simulink model "SecRwRtStHdrstUpwdDnwdIsPosChk"  (R2024b)
settings: Solver=FixedStepDiscrete  StartTime=0.0  StopTime=10.0  FixedStep=0.01  RelTol=1e-3
undefined symbols (not defined in the file or in its folder): KeSMSuSecRwStHeadrestUpwdDwnwdPosDelta_Val, KeSMSuSecRwStHeadrestUpwdDwnwdPosTolr_Val
libraries: StIsPosChkLib x9, simulink x5
settings Model: Creator=sn2xws  LastModifiedBy=sn55gm
settings Model: ModifiedHistory=|
  | 2023.8.1 V2.0.0 CR401790 增加模式21-26
  | V2.1.0
  | 2023.9.14  Bug 540886 修改模式判断到位的条件为10ms周期计算
  | Bug 541373 Md24到位置修改为常数1代表到位置
settings SolverCC: AlgebraicLoopSolver=TrustRegion
settings DataIOCC: SaveFormat=StructureWithTime  ReturnWorkspaceOutputs=off
settings OptimizationCC: DefaultParameterBehavior=Inlined  EnhancedBackFolding=on  PassReuseOutputArgsAs=Individual arguments  ZeroExternalMemoryAtStartup=off  ZeroInternalMemoryAtStartup=off  OptimizeBlockOrder=speed  DifferentSizesBufferReuse=on  OptimizationCustomize=off  EfficientTunableParamExpr=on
settings DebuggingCC: ParameterTunabilityLossMsg=error  UnconnectedInputMsg=warning  UnconnectedOutputMsg=warning  UnconnectedLineMsg=warning  ArithmeticOperatorsInVariantConditions=warning
settings ModelReferenceCC: EnableRefExpFcnMdlSchedulingChecks=on  ModelReferenceNumInstancesAllowed=Single
settings SFSimCC: MATLABDynamicMemAlloc=off  CustomCodeUndefinedFunction=UseInterfaceOnly
settings RTWCC: Description=AUTOSAR  SystemTargetFile=autosar.tlc  GenCodeOnly=on  TemplateMakefile=ert_default_tmf  GenerateReport=on  IncludeHyperlinkInReport=on  LaunchReport=on  DataTypeReplacement=CDataTypesFixedWidth  GenerateTraceInfo=on  GenerateTraceReport=on  GenerateTraceReportSl=on  GenerateTraceReportSf=on  GenerateTraceReportEml=on  GPUComputeCapability=3.5
settings CodeAppCC: ForceParamTrailComments=on  IgnoreCustomStorageClasses=off  OperatorAnnotations=on  SimulinkDataObjDesc=on  SFDataObjDesc=on  InsertBlockDesc=on
settings STFCustomTargetCC: TargetLangStandard=C99 (ISO)  MultiwordLength=256  ParMdlRefBuildCompliant=on  CompOptLevelCompliant=on  IncludeMdlTerminateFcn=off  CombineOutputUpdateFcns=on  SuppressErrorStatus=on  ERTCustomFileBanners=on  SupportNonFinite=off  SupportComplex=off  SupportContinuousTime=off  SupportNonInlinedSFcns=off  RemoveResetFunc=on  MATLABClassNameForMDSCustomization=Simulink.SoftwareTarget.ERTCustomization  AutosarCompliant=on  UseToolchainInfoCompliant=on  LookupTableObjectStructAxisOrder=2,1,3,4,...  LUTObjectStructOrderEvenSpacing=Size,Table,Breakpoints  SystemTargetFile=autosar.tlc
settings ERTTargetCC: TargetLangStandard=C99 (ISO)  ConcurrentExecutionCompliant=off  IncludeMdlTerminateFcn=off  SuppressErrorStatus=on  SupportNonFinite=off  SupportComplex=off  ModelStepFunctionPrototypeControlCompliant=off  CPPClassGenCompliant=off  AutosarCompliant=on  LookupTableObjectStructAxisOrder=2,1,3,4,...  LUTObjectStructOrderEvenSpacing=Size,Table,Breakpoints  ERTCustomFileTemplate=example_file_process.tlc  ERTFilePackagingFormat=Compact  BooleanTrueId=TRUE  BooleanFalseId=FALSE  DynamicArrayContainerType=coder::array

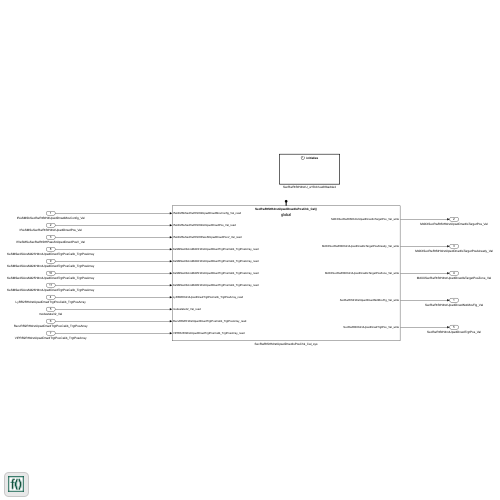
[thumbnail: Simulink's stored preview of the top-level diagram]
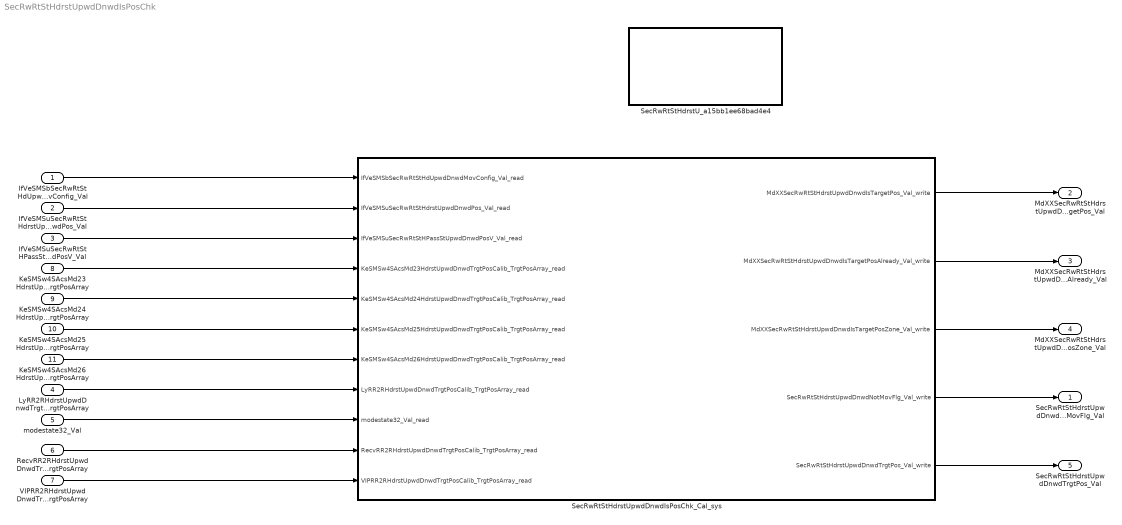
== system SecRwRtStHdrstUpwdDnwdIsPosChk ==
  IfVeSMSbSecRwRtStHdUpwdDnwdMovConfig_Val : Inport  OutDataTypeStr=boolean  PortDimensions=1
  IfVeSMSuSecRwRtStHdrstUpwdDnwdPos_Val : Inport  Port=2  OutDataTypeStr=uint16  PortDimensions=1
  IfVeSMSuSecRwRtStHPassStUpwdDnwdPosV_Val : Inport  Port=3  OutDataTypeStr=boolean  PortDimensions=1
  LyRR2RHdrstUpwdDnwdTrgtPosCalib_TrgtPosArray : Inport  Description=|  Port=4  OutDataTypeStr=uint16  PortDimensions=3
      | 0:Pos
      | 1:Max
      | 2:Min
  modestate32_Val : Inport  Port=5  OutDataTypeStr=uint32  PortDimensions=1
  RecvRR2RHdrstUpwdDnwdTrgtPosCalib_TrgtPosArray : Inport  Description=|  Port=6  OutDataTypeStr=uint16  PortDimensions=3
      | 0:Pos
      | 1:Max
      | 2:Min
  VIPRR2RHdrstUpwdDnwdTrgtPosCalib_TrgtPosArray : Inport  Description=|  Port=7  OutDataTypeStr=uint16  PortDimensions=3
      | 0:Pos
      | 1:Max
      | 2:Min
  KeSMSw4SAcsMd23HdrstUpwdDnwdTrgtPosCalib_TrgtPosArray : Inport  Description=|  Port=8  OutDataTypeStr=uint16  PortDimensions=3
      | 0:Pos
      | 1:Max
      | 2:Min
  KeSMSw4SAcsMd24HdrstUpwdDnwdTrgtPosCalib_TrgtPosArray : Inport  Description=|  Port=9  OutDataTypeStr=uint16  PortDimensions=3
      | 0:Pos
      | 1:Max
      | 2:Min
  KeSMSw4SAcsMd25HdrstUpwdDnwdTrgtPosCalib_TrgtPosArray : Inport  Description=|  Port=10  OutDataTypeStr=uint16  PortDimensions=3
      | 0:Pos
      | 1:Max
      | 2:Min
  KeSMSw4SAcsMd26HdrstUpwdDnwdTrgtPosCalib_TrgtPosArray : Inport  Description=|  Port=11  OutDataTypeStr=uint16  PortDimensions=3
      | 0:Pos
      | 1:Max
      | 2:Min
  SecRwRtStHdrstU_a15bb1ee68bad4e4 : Subsystem
  SecRwRtStHdrstUpwdDnwdIsPosChk_Cal_sys : Subsystem
  SecRwRtStHdrstUpwdDnwdNotMovFlg_Val : Outport  OutDataTypeStr=boolean  PortDimensions=1  VectorParamsAs1DForOutWhenUnconnected=off
  MdXXSecRwRtStHdrstUpwdDnwdIsTargetPos_Val : Outport  Port=2  OutDataTypeStr=uint32  PortDimensions=1  VectorParamsAs1DForOutWhenUnconnected=off
  MdXXSecRwRtStHdrstUpwdDnwdIsTargetPosAlready_Val : Outport  Port=3  OutDataTypeStr=uint32  PortDimensions=1  VectorParamsAs1DForOutWhenUnconnected=off
  MdXXSecRwRtStHdrstUpwdDnwdIsTargetPosZone_Val : Outport  Port=4  OutDataTypeStr=uint32  PortDimensions=1  VectorParamsAs1DForOutWhenUnconnected=off
  SecRwRtStHdrstUpwdDnwdTrgtPos_Val : Outport  Port=5  OutDataTypeStr=uint16  PortDimensions=1  VectorParamsAs1DForOutWhenUnconnected=off
  wires:
  IfVeSMSbSecRwRtStHdUpwdDnwdMovConfig_Val/1 -> SecRwRtStHdrstUpwdDnwdIsPosChk_Cal_sys/1(IfVeSMSbSecRwRtStHdUpwdDnwdMovConfig_Val_read)
  IfVeSMSuSecRwRtStHdrstUpwdDnwdPos_Val/1 -> SecRwRtStHdrstUpwdDnwdIsPosChk_Cal_sys/2(IfVeSMSuSecRwRtStHdrstUpwdDnwdPos_Val_read)
  IfVeSMSuSecRwRtStHPassStUpwdDnwdPosV_Val/1 -> SecRwRtStHdrstUpwdDnwdIsPosChk_Cal_sys/3(IfVeSMSuSecRwRtStHPassStUpwdDnwdPosV_Val_read)
  LyRR2RHdrstUpwdDnwdTrgtPosCalib_TrgtPosArray/1 -> SecRwRtStHdrstUpwdDnwdIsPosChk_Cal_sys/8(LyRR2RHdrstUpwdDnwdTrgtPosCalib_TrgtPosArray_read)
  modestate32_Val/1 -> SecRwRtStHdrstUpwdDnwdIsPosChk_Cal_sys/9(modestate32_Val_read)
  RecvRR2RHdrstUpwdDnwdTrgtPosCalib_TrgtPosArray/1 -> SecRwRtStHdrstUpwdDnwdIsPosChk_Cal_sys/10(RecvRR2RHdrstUpwdDnwdTrgtPosCalib_TrgtPosArray_read)
  VIPRR2RHdrstUpwdDnwdTrgtPosCalib_TrgtPosArray/1 -> SecRwRtStHdrstUpwdDnwdIsPosChk_Cal_sys/11(VIPRR2RHdrstUpwdDnwdTrgtPosCalib_TrgtPosArray_read)
  SecRwRtStHdrstUpwdDnwdIsPosChk_Cal_sys/1(MdXXSecRwRtStHdrstUpwdDnwdIsTargetPos_Val_write) -> MdXXSecRwRtStHdrstUpwdDnwdIsTargetPos_Val/1
  SecRwRtStHdrstUpwdDnwdIsPosChk_Cal_sys/2(MdXXSecRwRtStHdrstUpwdDnwdIsTargetPosAlready_Val_write) -> MdXXSecRwRtStHdrstUpwdDnwdIsTargetPosAlready_Val/1
  SecRwRtStHdrstUpwdDnwdIsPosChk_Cal_sys/3(MdXXSecRwRtStHdrstUpwdDnwdIsTargetPosZone_Val_write) -> MdXXSecRwRtStHdrstUpwdDnwdIsTargetPosZone_Val/1
  SecRwRtStHdrstUpwdDnwdIsPosChk_Cal_sys/4(SecRwRtStHdrstUpwdDnwdNotMovFlg_Val_write) -> SecRwRtStHdrstUpwdDnwdNotMovFlg_Val/1
  SecRwRtStHdrstUpwdDnwdIsPosChk_Cal_sys/5(SecRwRtStHdrstUpwdDnwdTrgtPos_Val_write) -> SecRwRtStHdrstUpwdDnwdTrgtPos_Val/1
  KeSMSw4SAcsMd23HdrstUpwdDnwdTrgtPosCalib_TrgtPosArray/1 -> SecRwRtStHdrstUpwdDnwdIsPosChk_Cal_sys/4(KeSMSw4SAcsMd23HdrstUpwdDnwdTrgtPosCalib_TrgtPosArray_read)
  KeSMSw4SAcsMd24HdrstUpwdDnwdTrgtPosCalib_TrgtPosArray/1 -> SecRwRtStHdrstUpwdDnwdIsPosChk_Cal_sys/5(KeSMSw4SAcsMd24HdrstUpwdDnwdTrgtPosCalib_TrgtPosArray_read)
  KeSMSw4SAcsMd25HdrstUpwdDnwdTrgtPosCalib_TrgtPosArray/1 -> SecRwRtStHdrstUpwdDnwdIsPosChk_Cal_sys/6(KeSMSw4SAcsMd25HdrstUpwdDnwdTrgtPosCalib_TrgtPosArray_read)
  KeSMSw4SAcsMd26HdrstUpwdDnwdTrgtPosCalib_TrgtPosArray/1 -> SecRwRtStHdrstUpwdDnwdIsPosChk_Cal_sys/7(KeSMSw4SAcsMd26HdrstUpwdDnwdTrgtPosCalib_TrgtPosArray_read)

== system SecRwRtStHdrstUpwdDnwdIsPosChk/SecRwRtStHdrstU_a15bb1ee68bad4e4 ==
  Event Listener : EventListener  EventName=reset

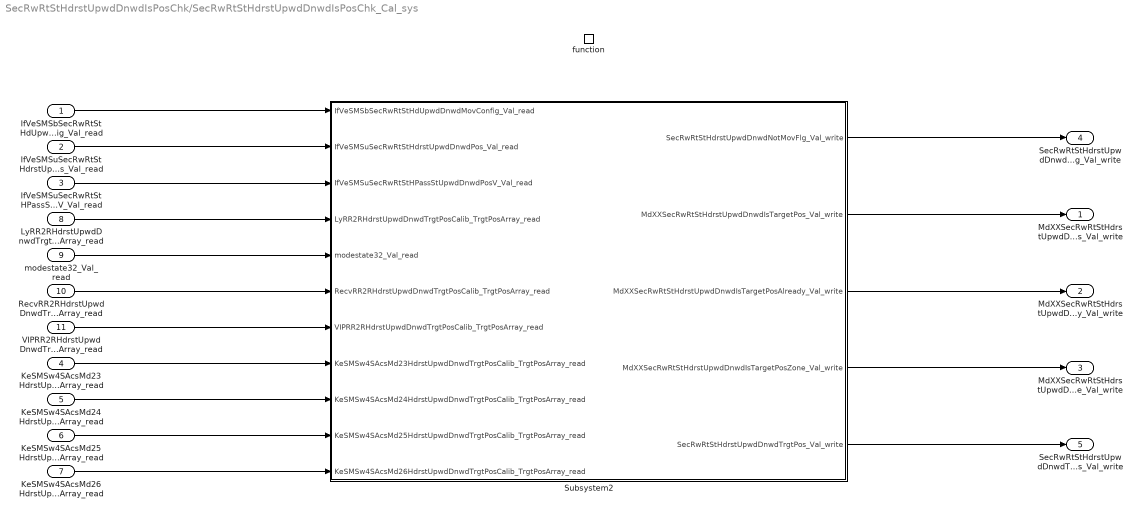
== system SecRwRtStHdrstUpwdDnwdIsPosChk/SecRwRtStHdrstUpwdDnwdIsPosChk_Cal_sys ==
  IfVeSMSbSecRwRtStHdUpwdDnwdMovConfig_Val_read : Inport
  IfVeSMSuSecRwRtStHdrstUpwdDnwdPos_Val_read : Inport  Port=2
  IfVeSMSuSecRwRtStHPassStUpwdDnwdPosV_Val_read : Inport  Port=3
  KeSMSw4SAcsMd23HdrstUpwdDnwdTrgtPosCalib_TrgtPosArray_read : Inport  Port=4
  KeSMSw4SAcsMd24HdrstUpwdDnwdTrgtPosCalib_TrgtPosArray_read : Inport  Port=5
  KeSMSw4SAcsMd25HdrstUpwdDnwdTrgtPosCalib_TrgtPosArray_read : Inport  Port=6
  KeSMSw4SAcsMd26HdrstUpwdDnwdTrgtPosCalib_TrgtPosArray_read : Inport  Port=7
  LyRR2RHdrstUpwdDnwdTrgtPosCalib_TrgtPosArray_read : Inport  Port=8
  modestate32_Val_read : Inport  Port=9
  RecvRR2RHdrstUpwdDnwdTrgtPosCalib_TrgtPosArray_read : Inport  Port=10
  VIPRR2RHdrstUpwdDnwdTrgtPosCalib_TrgtPosArray_read : Inport  Port=11
  function : TriggerPort  TriggerType=function-call  IsSimulinkFunction=on  FunctionName=SecRwRtStHdrstUpwdDnwdIsPosChk_Cal  VariantControl=(inherit)
  Subsystem2 : Subsystem
  MdXXSecRwRtStHdrstUpwdDnwdIsTargetPos_Val_write : Outport  VectorParamsAs1DForOutWhenUnconnected=off
      settings: EnsureOutportIsVirtual=on
  MdXXSecRwRtStHdrstUpwdDnwdIsTargetPosAlready_Val_write : Outport  Port=2  VectorParamsAs1DForOutWhenUnconnected=off
      settings: EnsureOutportIsVirtual=on
  MdXXSecRwRtStHdrstUpwdDnwdIsTargetPosZone_Val_write : Outport  Port=3  VectorParamsAs1DForOutWhenUnconnected=off
      settings: EnsureOutportIsVirtual=on
  SecRwRtStHdrstUpwdDnwdNotMovFlg_Val_write : Outport  Port=4  VectorParamsAs1DForOutWhenUnconnected=off
      settings: EnsureOutportIsVirtual=on
  SecRwRtStHdrstUpwdDnwdTrgtPos_Val_write : Outport  Port=5  VectorParamsAs1DForOutWhenUnconnected=off
      settings: EnsureOutportIsVirtual=on
  wires:
  LyRR2RHdrstUpwdDnwdTrgtPosCalib_TrgtPosArray_read/1 -> Subsystem2/4(LyRR2RHdrstUpwdDnwdTrgtPosCalib_TrgtPosArray_read)
  modestate32_Val_read/1 -> Subsystem2/5(modestate32_Val_read)
  RecvRR2RHdrstUpwdDnwdTrgtPosCalib_TrgtPosArray_read/1 -> Subsystem2/6(RecvRR2RHdrstUpwdDnwdTrgtPosCalib_TrgtPosArray_read)
  VIPRR2RHdrstUpwdDnwdTrgtPosCalib_TrgtPosArray_read/1 -> Subsystem2/7(VIPRR2RHdrstUpwdDnwdTrgtPosCalib_TrgtPosArray_read)
  KeSMSw4SAcsMd23HdrstUpwdDnwdTrgtPosCalib_TrgtPosArray_read/1 -> Subsystem2/8(KeSMSw4SAcsMd23HdrstUpwdDnwdTrgtPosCalib_TrgtPosArray_read)
  IfVeSMSuSecRwRtStHPassStUpwdDnwdPosV_Val_read/1 -> Subsystem2/3(IfVeSMSuSecRwRtStHPassStUpwdDnwdPosV_Val_read)
  KeSMSw4SAcsMd24HdrstUpwdDnwdTrgtPosCalib_TrgtPosArray_read/1 -> Subsystem2/9(KeSMSw4SAcsMd24HdrstUpwdDnwdTrgtPosCalib_TrgtPosArray_read)
  KeSMSw4SAcsMd25HdrstUpwdDnwdTrgtPosCalib_TrgtPosArray_read/1 -> Subsystem2/10(KeSMSw4SAcsMd25HdrstUpwdDnwdTrgtPosCalib_TrgtPosArray_read)
  IfVeSMSuSecRwRtStHdrstUpwdDnwdPos_Val_read/1 -> Subsystem2/2(IfVeSMSuSecRwRtStHdrstUpwdDnwdPos_Val_read)
  KeSMSw4SAcsMd26HdrstUpwdDnwdTrgtPosCalib_TrgtPosArray_read/1 -> Subsystem2/11(KeSMSw4SAcsMd26HdrstUpwdDnwdTrgtPosCalib_TrgtPosArray_read)
  IfVeSMSbSecRwRtStHdUpwdDnwdMovConfig_Val_read/1 -> Subsystem2/1(IfVeSMSbSecRwRtStHdUpwdDnwdMovConfig_Val_read)
  Subsystem2/1(SecRwRtStHdrstUpwdDnwdNotMovFlg_Val_write) -> SecRwRtStHdrstUpwdDnwdNotMovFlg_Val_write/1
  Subsystem2/2(MdXXSecRwRtStHdrstUpwdDnwdIsTargetPos_Val_write) -> MdXXSecRwRtStHdrstUpwdDnwdIsTargetPos_Val_write/1
  Subsystem2/3(MdXXSecRwRtStHdrstUpwdDnwdIsTargetPosAlready_Val_write) -> MdXXSecRwRtStHdrstUpwdDnwdIsTargetPosAlready_Val_write/1
  Subsystem2/4(MdXXSecRwRtStHdrstUpwdDnwdIsTargetPosZone_Val_write) -> MdXXSecRwRtStHdrstUpwdDnwdIsTargetPosZone_Val_write/1
  Subsystem2/5(SecRwRtStHdrstUpwdDnwdTrgtPos_Val_write) -> SecRwRtStHdrstUpwdDnwdTrgtPos_Val_write/1

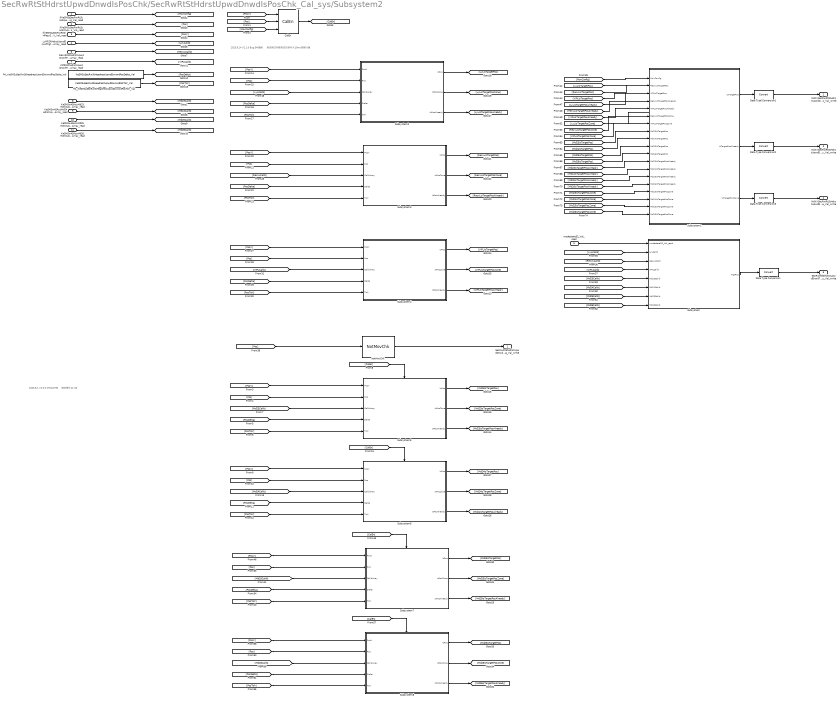
== system SecRwRtStHdrstUpwdDnwdIsPosChk/SecRwRtStHdrstUpwdDnwdIsPosChk_Cal_sys/Subsystem2 ==
  note: 2023.9.14 V2.1.0 Bug 540886 修改模式判断到位的条件为10ms周期计算
  note: 2023.8.1 V2.0.0 CR401790 增加模式21-26
  IfVeSMSbSecRwRtStHdUpwdDnwdMovConfig_Val_read : Inport
  IfVeSMSuSecRwRtStHdrstUpwdDnwdPos_Val_read : Inport  Port=2
  IfVeSMSuSecRwRtStHPassStUpwdDnwdPosV_Val_read : Inport  Port=3
  LyRR2RHdrstUpwdDnwdTrgtPosCalib_TrgtPosArray_read : Inport  Port=4
  modestate32_Val_read : Inport  Port=5
  RecvRR2RHdrstUpwdDnwdTrgtPosCalib_TrgtPosArray_read : Inport  Port=6
  VIPRR2RHdrstUpwdDnwdTrgtPosCalib_TrgtPosArray_read : Inport  Port=7
  KeSMSw4SAcsMd23HdrstUpwdDnwdTrgtPosCalib_TrgtPosArray_read : Inport  Port=8
  KeSMSw4SAcsMd24HdrstUpwdDnwdTrgtPosCalib_TrgtPosArray_read : Inport  Port=9
  KeSMSw4SAcsMd25HdrstUpwdDnwdTrgtPosCalib_TrgtPosArray_read : Inport  Port=10
  KeSMSw4SAcsMd26HdrstUpwdDnwdTrgtPosCalib_TrgtPosArray_read : Inport  Port=11
  CalEn : StIsPosChkLib/CalEn  SystemSampleTime=-1  VariantActivationTime=update diagram  AllowFlexibleInterface=on  Latency=0  AutoFrameSizeCalculation=off
  Data Type Conversion{,1..3} (4 alike) : DataTypeConversion  SaturateOnIntegerOverflow=off  RndMeth=Floor
  NotMovChk : StIsPosChkLib/NotMovChk  SystemSampleTime=-1  VariantActivationTime=update diagram  AllowFlexibleInterface=on  Latency=0  AutoFrameSizeCalculation=off
  PA_KeSMSuSecRwStHeadrestUpwdDwnwdPosDelta_Val : Constant  Value=KeSMSuSecRwStHeadrestUpwdDwnwdPosDelta_Val
  PA_KeSMSuSecRwStHeadrestUpwdDwnwdPosTolr_Val : Constant  Value=KeSMSuSecRwStHeadrestUpwdDwnwdPosTolr_Val
  Subsystem : Subsystem
  Subsystem1 : Subsystem
  Subsystem2 : Subsystem
  Subsystem3 : Subsystem
  Subsystem4 : Subsystem
  Subsystem5 : Subsystem
  Subsystem6 : Subsystem
  Subsystem7 : Subsystem
  Subsystem8 : Subsystem
  SecRwRtStHdrstUpwdDnwdNotMovFlg_Val_write : Outport  VectorParamsAs1DForOutWhenUnconnected=off
      settings: EnsureOutportIsVirtual=on
  MdXXSecRwRtStHdrstUpwdDnwdIsTargetPos_Val_write : Outport  Port=2  VectorParamsAs1DForOutWhenUnconnected=off
      settings: EnsureOutportIsVirtual=on
  MdXXSecRwRtStHdrstUpwdDnwdIsTargetPosAlready_Val_write : Outport  Port=3  VectorParamsAs1DForOutWhenUnconnected=off
      settings: EnsureOutportIsVirtual=on
  MdXXSecRwRtStHdrstUpwdDnwdIsTargetPosZone_Val_write : Outport  Port=4  VectorParamsAs1DForOutWhenUnconnected=off
      settings: EnsureOutportIsVirtual=on
  SecRwRtStHdrstUpwdDnwdTrgtPos_Val_write : Outport  Port=5  VectorParamsAs1DForOutWhenUnconnected=off
      settings: EnsureOutportIsVirtual=on
  wires:
  [VIPLIsTargetPosAlready] -> Subsystem1/5(VIPLIsTargetPosAlready)
  [Pos] -> NotMovChk/1
  PA_KeSMSuSecRwStHeadrestUpwdDwnwdPosTolr_Val/1 -> [PosTolr]
  [PosV] -> Subsystem2/1(PosV)
  [VIPLIsTargetPosZone] -> Subsystem1/7(VIPLIsTargetPosZone)
  modestate32_Val_read/1 -> Subsystem/1(modestate32_Val_read)
  NotMovChk/1 -> SecRwRtStHdrstUpwdDnwdNotMovFlg_Val_write/1
  Subsystem2/3(IsPosAlready) -> [LyLIsTargetPosAlready]
  [PosV] -> Subsystem3/1(PosV)
  [PosDelta] -> Subsystem3/4(Delta)
  [RecvLIsTargetPosZone] -> Subsystem1/6(RecvLIsTargetPosZone)
  Subsystem2/1(IsPos) -> [LyLIsTargetPos]
  [LyLIsTargetPosAlready] -> ?
  [PosDelta] -> Subsystem2/4(Delta)
  LyRR2RHdrstUpwdDnwdTrgtPosCalib_TrgtPosArray_read/1 -> [LyLCalib]
  RecvRR2RHdrstUpwdDnwdTrgtPosCalib_TrgtPosArray_read/1 -> [RecvLCalib]
  [PosV] -> Subsystem4/1(PosV)
  Subsystem4/2(IsPosZone) -> [VIPLIsTargetPosZone]
  Subsystem3/3(IsPosAlready) -> [RecvLIsTargetPosAlready]
  [VIPLCalib] -> Subsystem/4(VIPLCalib)
  [PosTolr] -> Subsystem3/5(Tolr)
  Data Type Conversion2/1 -> MdXXSecRwRtStHdrstUpwdDnwdIsTargetPosAlready_Val_write/1
  Subsystem1/1(IsTargetPos) -> Data Type Conversion1/1
  Subsystem4/1(IsPos) -> [VIPLIsTargetPos]
  VIPRR2RHdrstUpwdDnwdTrgtPosCalib_TrgtPosArray_read/1 -> [VIPLCalib]
  [Pos] -> Subsystem2/2(Pos)
  Subsystem3/2(IsPosZone) -> [RecvLIsTargetPosZone]
  PA_KeSMSuSecRwStHeadrestUpwdDwnwdPosDelta_Val/1 -> [PosDelta]
  [RecvLIsTargetPos] -> Subsystem1/2(RecvLIsTargetPos)
  Subsystem1/2(IsTargetPosAlready) -> Data Type Conversion2/1
  [LyLIsTargetPosZone] -> ?
  [PosTolr] -> Subsystem4/5(Tolr)
  CalEn/1 -> [CalEn]
  Subsystem/1(TrgtPos) -> Data Type Conversion/1
  Subsystem3/1(IsPos) -> [RecvLIsTargetPos]
  [RecvLCalib] -> Subsystem/3(RecvLCalib)
  [PosV] -> CalEn/1
  Subsystem4/3(IsPosAlready) -> [VIPLIsTargetPosAlready]
  [RecvLCalib] -> Subsystem3/3(CalibArray)
  Data Type Conversion1/1 -> MdXXSecRwRtStHdrstUpwdDnwdIsTargetPos_Val_write/1
  [MovConfig] -> Subsystem1/1(MovConfig)
  IfVeSMSuSecRwRtStHPassStUpwdDnwdPosV_Val_read/1 -> [PosV]
  [PosTolr] -> Subsystem2/5(Tolr)
  Subsystem2/2(IsPosZone) -> [LyLIsTargetPosZone]
  [Pos] -> Subsystem4/2(Pos)
  IfVeSMSbSecRwRtStHdUpwdDnwdMovConfig_Val_read/1 -> [MovConfig]
  [RecvLIsTargetPosAlready] -> Subsystem1/4(RecvLIsTargetPosAlready)
  Subsystem1/3(IsTargetPosZone) -> Data Type Conversion3/1
  [VIPLIsTargetPos] -> Subsystem1/3(VIPLIsTargetPos)
  [PosDelta] -> Subsystem4/4(Delta)
  [VIPLCalib] -> Subsystem4/3(CalibArray)
  [Pos] -> CalEn/2
  IfVeSMSuSecRwRtStHdrstUpwdDnwdPos_Val_read/1 -> [Pos]
  [LyLCalib] -> Subsystem2/3(CalibArray)
  [LyLCalib] -> Subsystem/2(LyLCalib)
  [Pos] -> Subsystem3/2(Pos)
  [MovConfig] -> CalEn/3
  Data Type Conversion3/1 -> MdXXSecRwRtStHdrstUpwdDnwdIsTargetPosZone_Val_write/1
  Data Type Conversion/1 -> SecRwRtStHdrstUpwdDnwdTrgtPos_Val_write/1
  [LyLIsTargetPos] -> ?
  KeSMSw4SAcsMd23HdrstUpwdDnwdTrgtPosCalib_TrgtPosArray_read/1 -> [Md23Calib]
  KeSMSw4SAcsMd24HdrstUpwdDnwdTrgtPosCalib_TrgtPosArray_read/1 -> [Md24Calib]
  KeSMSw4SAcsMd25HdrstUpwdDnwdTrgtPosCalib_TrgtPosArray_read/1 -> [Md25Calib]
  KeSMSw4SAcsMd26HdrstUpwdDnwdTrgtPosCalib_TrgtPosArray_read/1 -> [Md26Calib]
  [Md23Calib] -> Subsystem5/3(CalibArray)
  [PosDelta] -> Subsystem5/4(Delta)
  [Pos] -> Subsystem5/2(Pos)
  Subsystem5/3(IsPosAlready) -> [Md23IsTargetPosAlready]
  [PosTolr] -> Subsystem5/5(Tolr)
  Subsystem5/1(IsPos) -> [Md23IsTargetPos]
  Subsystem5/2(IsPosZone) -> [Md23IsTargetPosZone]
  [PosV] -> Subsystem5/1(PosV)
  [CalEn] -> Subsystem5/Enable
  [CalEn] -> Subsystem6/Enable
  [PosV] -> Subsystem6/1(PosV)
  Subsystem6/2(IsPosZone) -> [Md24IsTargetPosZone]
  Subsystem6/1(IsPos) -> [Md24IsTargetPos]
  [PosTolr] -> Subsystem6/5(Tolr)
  Subsystem6/3(IsPosAlready) -> [Md24IsTargetPosAlready]
  [Pos] -> Subsystem6/2(Pos)
  [PosDelta] -> Subsystem6/4(Delta)
  [Md24Calib] -> Subsystem6/3(CalibArray)
  [Md25Calib] -> Subsystem7/3(CalibArray)
  [PosDelta] -> Subsystem7/4(Delta)
  [Pos] -> Subsystem7/2(Pos)
  Subsystem7/3(IsPosAlready) -> [Md25IsTargetPosAlready]
  [PosTolr] -> Subsystem7/5(Tolr)
  Subsystem7/1(IsPos) -> [Md25IsTargetPos]
  Subsystem7/2(IsPosZone) -> [Md25IsTargetPosZone]
  [PosV] -> Subsystem7/1(PosV)
  [CalEn] -> Subsystem7/Enable
  [CalEn] -> Subsystem8/Enable
  [PosV] -> Subsystem8/1(PosV)
  Subsystem8/2(IsPosZone) -> [Md26IsTargetPosZone]
  Subsystem8/1(IsPos) -> [Md26IsTargetPos]
  [PosTolr] -> Subsystem8/5(Tolr)
  Subsystem8/3(IsPosAlready) -> [Md26IsTargetPosAlready]
  [Pos] -> Subsystem8/2(Pos)
  [PosDelta] -> Subsystem8/4(Delta)
  [Md26Calib] -> Subsystem8/3(CalibArray)
  [Md23Calib] -> Subsystem/5(Md23Calib)
  [Md24Calib] -> Subsystem/6(Md24Calib)
  [Md25Calib] -> Subsystem/7(Md25Calib)
  [Md26Calib] -> Subsystem/8(Md26Calib)
  [Md23IsTargetPos] -> Subsystem1/8(Md23IsTargetPos)
  [Md24IsTargetPos] -> Subsystem1/9(Md24IsTargetPos)
  [Md25IsTargetPos] -> Subsystem1/10(Md25IsTargetPos)
  [Md26IsTargetPos] -> Subsystem1/11(Md26IsTargetPos)
  [Md23IsTargetPosAlready] -> Subsystem1/12(Md23IsTargetPosAlready)
  [Md24IsTargetPosAlready] -> Subsystem1/13(Md24IsTargetPosAlready)
  [Md25IsTargetPosAlready] -> Subsystem1/14(Md25IsTargetPosAlready)
  [Md26IsTargetPosAlready] -> Subsystem1/15(Md26IsTargetPosAlready)
  [Md23IsTargetPosZone] -> Subsystem1/16(Md23IsTargetPosZone)
  [Md24IsTargetPosZone] -> Subsystem1/17(Md24IsTargetPosZone)
  [Md25IsTargetPosZone] -> Subsystem1/18(Md25IsTargetPosZone)
  [Md26IsTargetPosZone] -> Subsystem1/19(Md26IsTargetPosZone)

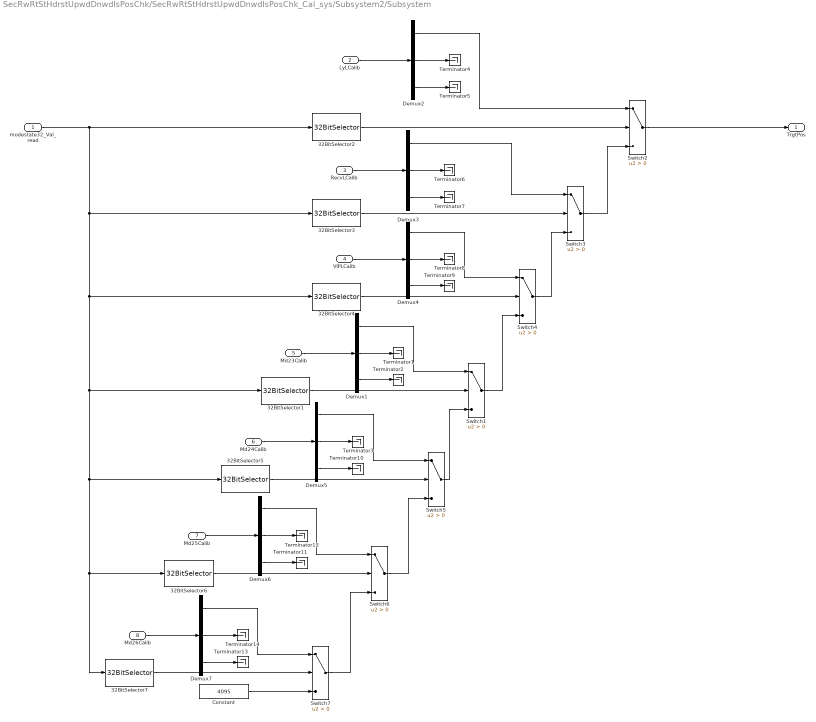
== system SecRwRtStHdrstUpwdDnwdIsPosChk/SecRwRtStHdrstUpwdDnwdIsPosChk_Cal_sys/Subsystem2/Subsystem ==
  modestate32_Val_read : Inport
  LyLCalib : Inport  Port=2
  RecvLCalib : Inport  Port=3
  VIPLCalib : Inport  Port=4
  Md23Calib : Inport  Port=5
  Md24Calib : Inport  Port=6
  Md25Calib : Inport  Port=7
  Md26Calib : Inport  Port=8
  32BitSelector1 : StIsPosChkLib/32BitSelector  BitNum=22
  32BitSelector2 : StIsPosChkLib/32BitSelector  BitNum=14
  32BitSelector3 : StIsPosChkLib/32BitSelector  BitNum=12
  32BitSelector4 : StIsPosChkLib/32BitSelector  BitNum=11
  32BitSelector5 : StIsPosChkLib/32BitSelector  BitNum=23
  32BitSelector6 : StIsPosChkLib/32BitSelector  BitNum=24
  32BitSelector7 : StIsPosChkLib/32BitSelector  BitNum=25
  Constant : Constant  Value=4095  OutDataTypeStr=uint16
  Demux{1..7} (7 alike) : Demux  Outputs=3
  Switch{1..7} (7 alike) : Switch  Criteria=u2 > Threshold  SaturateOnIntegerOverflow=off  InputSameDT=off
  Terminator{1..14} (14 alike) : Terminator
  TrgtPos : Outport  VectorParamsAs1DForOutWhenUnconnected=off
      settings: EnsureOutportIsVirtual=on
  wires:
  modestate32_Val_read/1 -> 32BitSelector2/1, 32BitSelector3/1, 32BitSelector7/1, 32BitSelector6/1, 32BitSelector5/1, 32BitSelector1/1, 32BitSelector4/1
  Switch2/1 -> TrgtPos/1
  Switch3/1 -> Switch2/3
  Switch4/1 -> Switch3/3
  32BitSelector2/1 -> Switch2/2
  32BitSelector3/1 -> Switch3/2
  32BitSelector4/1 -> Switch4/2
  Demux2/1 -> Switch2/1
  Demux2/3 -> Terminator5/1
  Demux2/2 -> Terminator4/1
  LyLCalib/1 -> Demux2/1
  RecvLCalib/1 -> Demux3/1
  Demux3/2 -> Terminator6/1
  Demux3/3 -> Terminator7/1
  Demux3/1 -> Switch3/1
  Demux4/1 -> Switch4/1
  Demux4/3 -> Terminator9/1
  Demux4/2 -> Terminator8/1
  VIPLCalib/1 -> Demux4/1
  Md23Calib/1 -> Demux1/1
  Demux1/2 -> Terminator1/1
  Demux1/3 -> Terminator2/1
  Demux1/1 -> Switch1/1
  32BitSelector1/1 -> Switch1/2
  Switch1/1 -> Switch4/3
  Switch5/1 -> Switch1/3
  32BitSelector5/1 -> Switch5/2
  Demux5/1 -> Switch5/1
  Demux5/3 -> Terminator10/1
  Demux5/2 -> Terminator3/1
  Md24Calib/1 -> Demux5/1
  Md25Calib/1 -> Demux6/1
  Demux6/2 -> Terminator12/1
  Demux6/3 -> Terminator11/1
  Demux6/1 -> Switch6/1
  32BitSelector6/1 -> Switch6/2
  Switch6/1 -> Switch5/3
  Switch7/1 -> Switch6/3
  32BitSelector7/1 -> Switch7/2
  Demux7/1 -> Switch7/1
  Demux7/3 -> Terminator13/1
  Demux7/2 -> Terminator14/1
  Md26Calib/1 -> Demux7/1
  Constant/1 -> Switch7/3

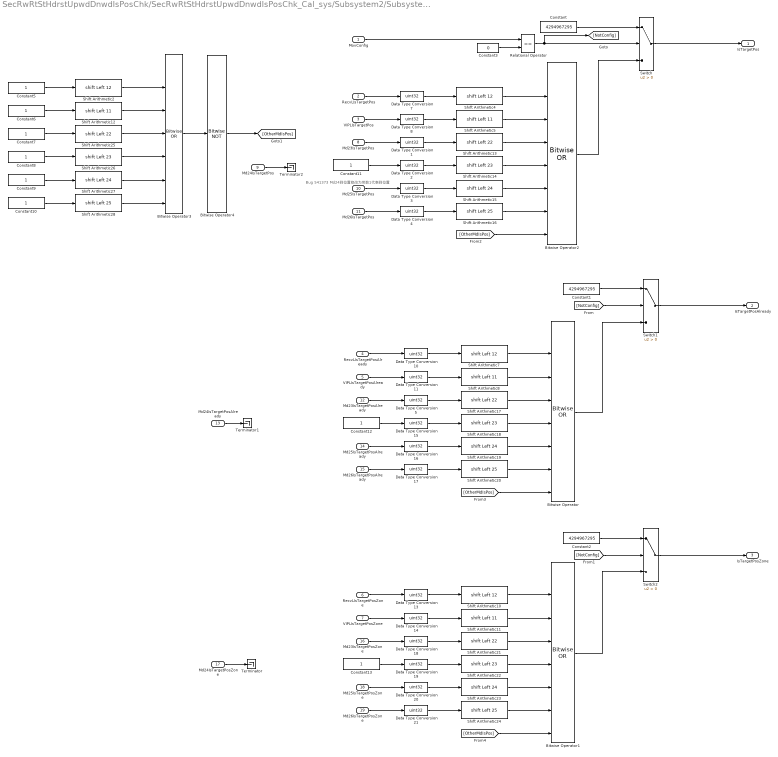
== system SecRwRtStHdrstUpwdDnwdIsPosChk/SecRwRtStHdrstUpwdDnwdIsPosChk_Cal_sys/Subsystem2/Subsystem1 ==
  note: Bug 541373 Md24到位置修改为常数1代表到位置
  MovConfig : Inport
  RecvLIsTargetPos : Inport  Port=2
  VIPLIsTargetPos : Inport  Port=3
  RecvLIsTargetPosAlready : Inport  Port=4
  VIPLIsTargetPosAlready : Inport  Port=5
  RecvLIsTargetPosZone : Inport  Port=6
  VIPLIsTargetPosZone : Inport  Port=7
  Md23IsTargetPos : Inport  Port=8
  Md24IsTargetPos : Inport  Port=9
  Md25IsTargetPos : Inport  Port=10
  Md26IsTargetPos : Inport  Port=11
  Md23IsTargetPosAlready : Inport  Port=12
  Md24IsTargetPosAlready : Inport  Port=13
  Md25IsTargetPosAlready : Inport  Port=14
  Md26IsTargetPosAlready : Inport  Port=15
  Md23IsTargetPosZone : Inport  Port=16
  Md24IsTargetPosZone : Inport  Port=17
  Md25IsTargetPosZone : Inport  Port=18
  Md26IsTargetPosZone : Inport  Port=19
  Bitwise Operator : simulink/Logic and Bit Operations/Bitwise Operator  logicop=OR  UseBitMask=off  NumInputPorts=8  BitMask=bin2dec('11011001')  BitMaskRealWorld=Stored Integer
  Bitwise Operator1 : simulink/Logic and Bit Operations/Bitwise Operator  logicop=OR  UseBitMask=off  NumInputPorts=8  BitMask=bin2dec('11011001')  BitMaskRealWorld=Stored Integer
  Bitwise Operator2 : simulink/Logic and Bit Operations/Bitwise Operator  logicop=OR  UseBitMask=off  NumInputPorts=8  BitMask=bin2dec('11011001')  BitMaskRealWorld=Stored Integer
  Bitwise Operator3 : simulink/Logic and Bit Operations/Bitwise Operator  logicop=OR  UseBitMask=off  NumInputPorts=7  BitMask=bin2dec('11011001')  BitMaskRealWorld=Stored Integer
  Bitwise Operator4 : simulink/Logic and Bit Operations/Bitwise Operator  logicop=NOT  UseBitMask=off  BitMask=bin2dec('11011001')  BitMaskRealWorld=Stored Integer
  Constant : Constant  Value=4294967295  OutDataTypeStr=uint32
  Constant1 : Constant  Value=4294967295  OutDataTypeStr=uint32
  Constant{5..13} (9 alike) : Constant  OutDataTypeStr=uint32
  Constant2 : Constant  Value=4294967295  OutDataTypeStr=uint32
  Constant3 : Constant  Value=0  OutDataTypeStr=uint8
  Data Type Conversion{1..5,7..8,10..11,13..21} (18 alike) : DataTypeConversion  OutDataTypeStr=uint32  SaturateOnIntegerOverflow=off  RndMeth=Floor
  Relational Operator : RelationalOperator  Operator===  OutDataTypeStr=boolean  RndMeth=Simplest  InputSameDT=off
  Shift Arithmetic{2,4,7,10} (4 alike) : ArithShift  BitShiftNumber=12  BitShiftDirection=Left
  Shift Arithmetic{5,8,11..12} (4 alike) : ArithShift  BitShiftNumber=11  BitShiftDirection=Left
  Shift Arithmetic{13,17,21,25} (4 alike) : ArithShift  BitShiftNumber=22  BitShiftDirection=Left
  Shift Arithmetic{14,18,22,26} (4 alike) : ArithShift  BitShiftNumber=23  BitShiftDirection=Left
  Shift Arithmetic{15,19,23,27} (4 alike) : ArithShift  BitShiftNumber=24  BitShiftDirection=Left
  Shift Arithmetic{16,20,24,28} (4 alike) : ArithShift  BitShiftNumber=25  BitShiftDirection=Left
  Switch : Switch  Criteria=u2 > Threshold  SaturateOnIntegerOverflow=off  InputSameDT=off
  Switch1 : Switch  Criteria=u2 > Threshold  SaturateOnIntegerOverflow=off  InputSameDT=off
  Switch2 : Switch  Criteria=u2 > Threshold  SaturateOnIntegerOverflow=off  InputSameDT=off
  Terminator : Terminator
  Terminator1 : Terminator
  Terminator2 : Terminator
  IsTargetPos : Outport  VectorParamsAs1DForOutWhenUnconnected=off
      settings: EnsureOutportIsVirtual=on
  IsTargetPosAlready : Outport  Port=2  VectorParamsAs1DForOutWhenUnconnected=off
      settings: EnsureOutportIsVirtual=on
  IsTargetPosZone : Outport  Port=3  VectorParamsAs1DForOutWhenUnconnected=off
      settings: EnsureOutportIsVirtual=on
  wires:
  Constant3/1 -> Relational Operator/2
  Constant/1 -> Switch/1
  Relational Operator/1 -> [NotConfig], Switch/2
  MovConfig/1 -> Relational Operator/1
  Switch/1 -> IsTargetPos/1
  [NotConfig] -> Switch1/2
  Constant1/1 -> Switch1/1
  Switch1/1 -> IsTargetPosAlready/1
  Switch2/1 -> IsTargetPosZone/1
  Constant2/1 -> Switch2/1
  [NotConfig] -> Switch2/2
  Bitwise Operator1/1 -> Switch2/3
  Bitwise Operator/1 -> Switch1/3
  Bitwise Operator2/1 -> Switch/3
  Shift Arithmetic4/1 -> Bitwise Operator2/2
  Shift Arithmetic5/1 -> Bitwise Operator2/3
  Data Type Conversion7/1 -> Shift Arithmetic4/1
  Data Type Conversion8/1 -> Shift Arithmetic5/1
  RecvLIsTargetPos/1 -> Data Type Conversion7/1
  VIPLIsTargetPos/1 -> Data Type Conversion8/1
  VIPLIsTargetPosAlready/1 -> Data Type Conversion11/1
  RecvLIsTargetPosAlready/1 -> Data Type Conversion10/1
  Data Type Conversion11/1 -> Shift Arithmetic8/1
  Data Type Conversion10/1 -> Shift Arithmetic7/1
  Shift Arithmetic8/1 -> Bitwise Operator/3
  Shift Arithmetic7/1 -> Bitwise Operator/2
  Data Type Conversion14/1 -> Shift Arithmetic11/1
  Data Type Conversion13/1 -> Shift Arithmetic10/1
  VIPLIsTargetPosZone/1 -> Data Type Conversion14/1
  Shift Arithmetic10/1 -> Bitwise Operator1/2
  RecvLIsTargetPosZone/1 -> Data Type Conversion13/1
  Shift Arithmetic11/1 -> Bitwise Operator1/3
  Constant6/1 -> Shift Arithmetic12/1
  Constant5/1 -> Shift Arithmetic2/1
  Shift Arithmetic12/1 -> Bitwise Operator3/3
  Shift Arithmetic2/1 -> Bitwise Operator3/2
  Bitwise Operator3/1 -> Bitwise Operator4/1
  Bitwise Operator4/1 -> [OtherMdIsPos]
  [OtherMdIsPos] -> Bitwise Operator2/8
  Md23IsTargetPos/1 -> Data Type Conversion1/1
  Data Type Conversion1/1 -> Shift Arithmetic13/1
  Shift Arithmetic13/1 -> Bitwise Operator2/4
  Shift Arithmetic14/1 -> Bitwise Operator2/5
  Data Type Conversion2/1 -> Shift Arithmetic14/1
  Md25IsTargetPos/1 -> Data Type Conversion3/1
  Data Type Conversion3/1 -> Shift Arithmetic15/1
  Shift Arithmetic15/1 -> Bitwise Operator2/6
  Data Type Conversion4/1 -> Shift Arithmetic16/1
  Md26IsTargetPos/1 -> Data Type Conversion4/1
  Shift Arithmetic16/1 -> Bitwise Operator2/7
  [OtherMdIsPos] -> Bitwise Operator/8
  Shift Arithmetic17/1 -> Bitwise Operator/4
  Data Type Conversion5/1 -> Shift Arithmetic17/1
  Md23IsTargetPosAlready/1 -> Data Type Conversion5/1
  Data Type Conversion15/1 -> Shift Arithmetic18/1
  Shift Arithmetic18/1 -> Bitwise Operator/5
  Shift Arithmetic19/1 -> Bitwise Operator/6
  Data Type Conversion16/1 -> Shift Arithmetic19/1
  Md25IsTargetPosAlready/1 -> Data Type Conversion16/1
  Md26IsTargetPosAlready/1 -> Data Type Conversion17/1
  Data Type Conversion17/1 -> Shift Arithmetic20/1
  Shift Arithmetic20/1 -> Bitwise Operator/7
  [OtherMdIsPos] -> Bitwise Operator1/8
  Shift Arithmetic21/1 -> Bitwise Operator1/4
  Md23IsTargetPosZone/1 -> Data Type Conversion18/1
  Data Type Conversion18/1 -> Shift Arithmetic21/1
  Data Type Conversion19/1 -> Shift Arithmetic22/1
  Shift Arithmetic22/1 -> Bitwise Operator1/5
  Shift Arithmetic23/1 -> Bitwise Operator1/6
  Md25IsTargetPosZone/1 -> Data Type Conversion20/1
  Data Type Conversion20/1 -> Shift Arithmetic23/1
  Data Type Conversion21/1 -> Shift Arithmetic24/1
  Md26IsTargetPosZone/1 -> Data Type Conversion21/1
  Shift Arithmetic24/1 -> Bitwise Operator1/7
  Shift Arithmetic25/1 -> Bitwise Operator3/4
  Constant7/1 -> Shift Arithmetic25/1
  Constant8/1 -> Shift Arithmetic26/1
  Shift Arithmetic26/1 -> Bitwise Operator3/5
  Shift Arithmetic27/1 -> Bitwise Operator3/6
  Constant9/1 -> Shift Arithmetic27/1
  Constant10/1 -> Shift Arithmetic28/1
  Shift Arithmetic28/1 -> Bitwise Operator3/7
  Md24IsTargetPosZone/1 -> Terminator/1
  Md24IsTargetPosAlready/1 -> Terminator1/1
  Md24IsTargetPos/1 -> Terminator2/1
  Constant11/1 -> Data Type Conversion2/1
  Constant12/1 -> Data Type Conversion15/1
  Constant13/1 -> Data Type Conversion19/1

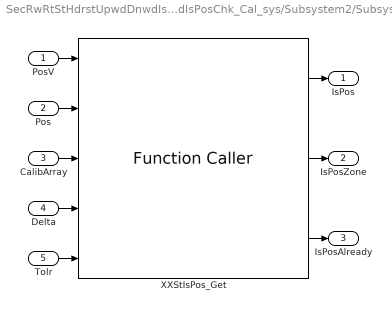
== system SecRwRtStHdrstUpwdDnwdIsPosChk/SecRwRtStHdrstUpwdDnwdIsPosChk_Cal_sys/Subsystem2/Subsystem2 ==
  PosV : Inport
  Pos : Inport  Port=2
  CalibArray : Inport  Port=3
  Delta : Inport  Port=4
  Tolr : Inport  Port=5
  XXStIsPos_Get : FunctionCaller  FunctionPrototype=[IsPos,IsPosZone,IsPosAlready] = XXStIsPos_Get(PosV,Pos,CalibArray,Delta,Tolr)  InputArgumentSpecifications=boolean(true), uint16(1), uint16([1;1;1]), uint16(1), uint16(1)  OutputArgumentSpecifications=boolean(true), boolean(true), boolean(true)
  IsPos : Outport  VectorParamsAs1DForOutWhenUnconnected=off
  IsPosZone : Outport  Port=2  VectorParamsAs1DForOutWhenUnconnected=off
  IsPosAlready : Outport  Port=3  VectorParamsAs1DForOutWhenUnconnected=off
  wires:
  PosV/1 -> XXStIsPos_Get/1
  XXStIsPos_Get/2 -> IsPosZone/1
  Pos/1 -> XXStIsPos_Get/2
  Delta/1 -> XXStIsPos_Get/4
  Tolr/1 -> XXStIsPos_Get/5
  XXStIsPos_Get/1 -> IsPos/1
  XXStIsPos_Get/3 -> IsPosAlready/1
  CalibArray/1 -> XXStIsPos_Get/3

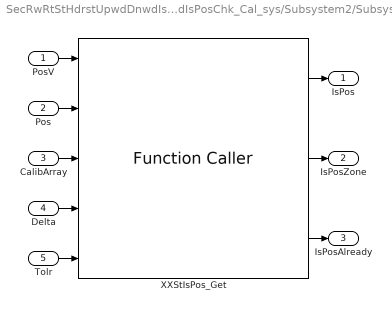
== system SecRwRtStHdrstUpwdDnwdIsPosChk/SecRwRtStHdrstUpwdDnwdIsPosChk_Cal_sys/Subsystem2/Subsystem3 ==
  PosV : Inport
  Pos : Inport  Port=2
  CalibArray : Inport  Port=3
  Delta : Inport  Port=4
  Tolr : Inport  Port=5
  XXStIsPos_Get : FunctionCaller  FunctionPrototype=[IsPos,IsPosZone,IsPosAlready] = XXStIsPos_Get(PosV,Pos,CalibArray,Delta,Tolr)  InputArgumentSpecifications=boolean(true), uint16(1), uint16([1;1;1]), uint16(1), uint16(1)  OutputArgumentSpecifications=boolean(true), boolean(true), boolean(true)
  IsPos : Outport  VectorParamsAs1DForOutWhenUnconnected=off
  IsPosZone : Outport  Port=2  VectorParamsAs1DForOutWhenUnconnected=off
  IsPosAlready : Outport  Port=3  VectorParamsAs1DForOutWhenUnconnected=off
  wires:
  PosV/1 -> XXStIsPos_Get/1
  XXStIsPos_Get/2 -> IsPosZone/1
  Pos/1 -> XXStIsPos_Get/2
  Delta/1 -> XXStIsPos_Get/4
  Tolr/1 -> XXStIsPos_Get/5
  XXStIsPos_Get/1 -> IsPos/1
  XXStIsPos_Get/3 -> IsPosAlready/1
  CalibArray/1 -> XXStIsPos_Get/3

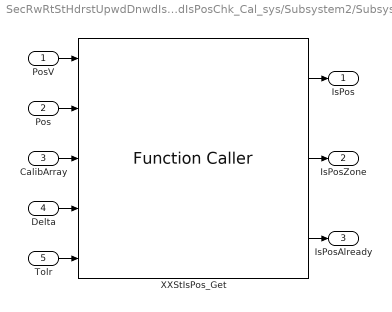
== system SecRwRtStHdrstUpwdDnwdIsPosChk/SecRwRtStHdrstUpwdDnwdIsPosChk_Cal_sys/Subsystem2/Subsystem4 ==
  PosV : Inport
  Pos : Inport  Port=2
  CalibArray : Inport  Port=3
  Delta : Inport  Port=4
  Tolr : Inport  Port=5
  XXStIsPos_Get : FunctionCaller  FunctionPrototype=[IsPos,IsPosZone,IsPosAlready] = XXStIsPos_Get(PosV,Pos,CalibArray,Delta,Tolr)  InputArgumentSpecifications=boolean(true), uint16(1), uint16([1;1;1]), uint16(1), uint16(1)  OutputArgumentSpecifications=boolean(true), boolean(true), boolean(true)
  IsPos : Outport  VectorParamsAs1DForOutWhenUnconnected=off
  IsPosZone : Outport  Port=2  VectorParamsAs1DForOutWhenUnconnected=off
  IsPosAlready : Outport  Port=3  VectorParamsAs1DForOutWhenUnconnected=off
  wires:
  PosV/1 -> XXStIsPos_Get/1
  XXStIsPos_Get/2 -> IsPosZone/1
  Pos/1 -> XXStIsPos_Get/2
  Delta/1 -> XXStIsPos_Get/4
  Tolr/1 -> XXStIsPos_Get/5
  XXStIsPos_Get/1 -> IsPos/1
  XXStIsPos_Get/3 -> IsPosAlready/1
  CalibArray/1 -> XXStIsPos_Get/3

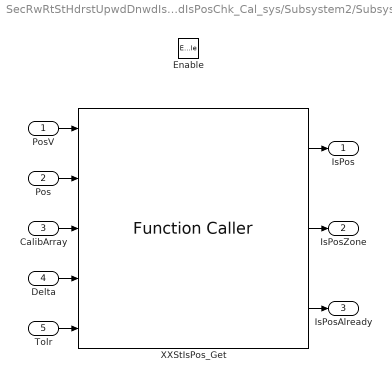
== system SecRwRtStHdrstUpwdDnwdIsPosChk/SecRwRtStHdrstUpwdDnwdIsPosChk_Cal_sys/Subsystem2/Subsystem5 ==
  PosV : Inport
  Pos : Inport  Port=2
  CalibArray : Inport  Port=3
  Delta : Inport  Port=4
  Tolr : Inport  Port=5
  Enable : EnablePort
  XXStIsPos_Get : FunctionCaller  FunctionPrototype=[IsPos,IsPosZone,IsPosAlready] = XXStIsPos_Get(PosV,Pos,CalibArray,Delta,Tolr)  InputArgumentSpecifications=boolean(true), uint16(1), uint16([1;1;1]), uint16(1), uint16(1)  OutputArgumentSpecifications=boolean(true), boolean(true), boolean(true)
  IsPos : Outport  VectorParamsAs1DForOutWhenUnconnected=off
  IsPosZone : Outport  Port=2  VectorParamsAs1DForOutWhenUnconnected=off
  IsPosAlready : Outport  Port=3  VectorParamsAs1DForOutWhenUnconnected=off
  wires:
  CalibArray/1 -> XXStIsPos_Get/3
  XXStIsPos_Get/3 -> IsPosAlready/1
  XXStIsPos_Get/1 -> IsPos/1
  Tolr/1 -> XXStIsPos_Get/5
  Delta/1 -> XXStIsPos_Get/4
  Pos/1 -> XXStIsPos_Get/2
  XXStIsPos_Get/2 -> IsPosZone/1
  PosV/1 -> XXStIsPos_Get/1

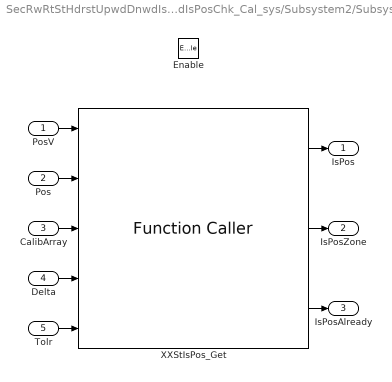
== system SecRwRtStHdrstUpwdDnwdIsPosChk/SecRwRtStHdrstUpwdDnwdIsPosChk_Cal_sys/Subsystem2/Subsystem6 ==
  PosV : Inport
  Pos : Inport  Port=2
  CalibArray : Inport  Port=3
  Delta : Inport  Port=4
  Tolr : Inport  Port=5
  Enable : EnablePort
  XXStIsPos_Get : FunctionCaller  FunctionPrototype=[IsPos,IsPosZone,IsPosAlready] = XXStIsPos_Get(PosV,Pos,CalibArray,Delta,Tolr)  InputArgumentSpecifications=boolean(true), uint16(1), uint16([1;1;1]), uint16(1), uint16(1)  OutputArgumentSpecifications=boolean(true), boolean(true), boolean(true)
  IsPos : Outport  VectorParamsAs1DForOutWhenUnconnected=off
  IsPosZone : Outport  Port=2  VectorParamsAs1DForOutWhenUnconnected=off
  IsPosAlready : Outport  Port=3  VectorParamsAs1DForOutWhenUnconnected=off
  wires:
  PosV/1 -> XXStIsPos_Get/1
  XXStIsPos_Get/2 -> IsPosZone/1
  Pos/1 -> XXStIsPos_Get/2
  Delta/1 -> XXStIsPos_Get/4
  Tolr/1 -> XXStIsPos_Get/5
  XXStIsPos_Get/1 -> IsPos/1
  XXStIsPos_Get/3 -> IsPosAlready/1
  CalibArray/1 -> XXStIsPos_Get/3

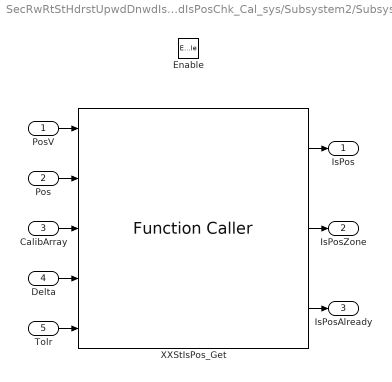
== system SecRwRtStHdrstUpwdDnwdIsPosChk/SecRwRtStHdrstUpwdDnwdIsPosChk_Cal_sys/Subsystem2/Subsystem7 ==
  PosV : Inport
  Pos : Inport  Port=2
  CalibArray : Inport  Port=3
  Delta : Inport  Port=4
  Tolr : Inport  Port=5
  Enable : EnablePort
  XXStIsPos_Get : FunctionCaller  FunctionPrototype=[IsPos,IsPosZone,IsPosAlready] = XXStIsPos_Get(PosV,Pos,CalibArray,Delta,Tolr)  InputArgumentSpecifications=boolean(true), uint16(1), uint16([1;1;1]), uint16(1), uint16(1)  OutputArgumentSpecifications=boolean(true), boolean(true), boolean(true)
  IsPos : Outport  VectorParamsAs1DForOutWhenUnconnected=off
  IsPosZone : Outport  Port=2  VectorParamsAs1DForOutWhenUnconnected=off
  IsPosAlready : Outport  Port=3  VectorParamsAs1DForOutWhenUnconnected=off
  wires:
  CalibArray/1 -> XXStIsPos_Get/3
  XXStIsPos_Get/3 -> IsPosAlready/1
  XXStIsPos_Get/1 -> IsPos/1
  Tolr/1 -> XXStIsPos_Get/5
  Delta/1 -> XXStIsPos_Get/4
  Pos/1 -> XXStIsPos_Get/2
  XXStIsPos_Get/2 -> IsPosZone/1
  PosV/1 -> XXStIsPos_Get/1

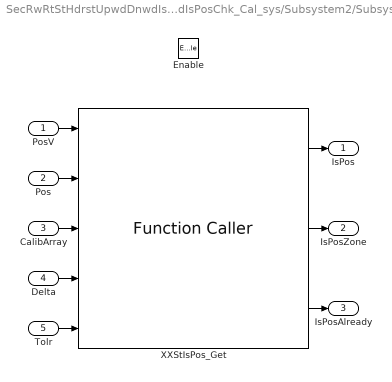
== system SecRwRtStHdrstUpwdDnwdIsPosChk/SecRwRtStHdrstUpwdDnwdIsPosChk_Cal_sys/Subsystem2/Subsystem8 ==
  PosV : Inport
  Pos : Inport  Port=2
  CalibArray : Inport  Port=3
  Delta : Inport  Port=4
  Tolr : Inport  Port=5
  Enable : EnablePort
  XXStIsPos_Get : FunctionCaller  FunctionPrototype=[IsPos,IsPosZone,IsPosAlready] = XXStIsPos_Get(PosV,Pos,CalibArray,Delta,Tolr)  InputArgumentSpecifications=boolean(true), uint16(1), uint16([1;1;1]), uint16(1), uint16(1)  OutputArgumentSpecifications=boolean(true), boolean(true), boolean(true)
  IsPos : Outport  VectorParamsAs1DForOutWhenUnconnected=off
  IsPosZone : Outport  Port=2  VectorParamsAs1DForOutWhenUnconnected=off
  IsPosAlready : Outport  Port=3  VectorParamsAs1DForOutWhenUnconnected=off
  wires:
  PosV/1 -> XXStIsPos_Get/1
  XXStIsPos_Get/2 -> IsPosZone/1
  Pos/1 -> XXStIsPos_Get/2
  Delta/1 -> XXStIsPos_Get/4
  Tolr/1 -> XXStIsPos_Get/5
  XXStIsPos_Get/1 -> IsPos/1
  XXStIsPos_Get/3 -> IsPosAlready/1
  CalibArray/1 -> XXStIsPos_Get/3
